simulink model "pointing_group24"  (R2023b)
settings: Solver=FixedStepAuto  StartTime=0.0  StopTime=T  RelTol=1e-3
values from neighbouring files (symbols this model uses):
  a = 6939    [Air_Drag_script.m]    (also in main.m = 6939.063; main_group24.m = 6978)
  AccMagn = 0.5    [main_group24.m]
  AccSunSens = 0.125    [main_group24.m]
  ARW = deg2rad(0.10)    [main_group24.m]
  by = 0.1    [main_group24.m]
  bz = 0.1    [main_group24.m]
  c = 2.99792*10^8    (= 299792000)    [main.m]    (also in main_group24.m = 299792458)
  Cd = 2.2    [main_group24.m]
  e = 0    [Air_Drag_script.m]    (also in main.m = 0.001304; main_group24.m)
  G = [gn, gm, gvali, gsvi]    [main.m]    (also in main_group24.m)
  GyroSampleRate = 10    [main_group24.m]
  H = [hn, hm, hvali, hsvi]    [main.m]    (also in main_group24.m)
  H_0 = ((g1_0^2)+(g1_1^2)+(h1_1^2))^0.5    (= 2.98059244128e-05)    [main_group24.m]
  i = deg2rad(97.5307)    [Air_Drag_script.m]    (also in main.m; main_group24.m = deg2rad(98))
  I_tot = [Ix 0 0; 0 Iy 0; 0 0 Iz]    [data_mass.m]    (also in main_group24.m)
  invI_tot = inv(I_tot)    [data_mass.m]    (also in main_group24.m)
  Ix = J(1,1)    [Air_Drag_script.m]    (also in data_mass.m = 0.0755003333333; main.m = 0.057749855; main_group24.m = 0.0755003333333)
  Iy = J(2,2)    [Air_Drag_script.m]    (also in data_mass.m = 0.0755003333333; main.m = 0.04143542; main_group24.m = 0.0755003333333)
  Iz = J(3,3)    [Air_Drag_script.m]    (also in data_mass.m = 0.055; main.m = 0.024624309; main_group24.m = 0.055)
  k1 = 5e-2    (= 0.05)    [main_group24.m]
  k2 = 2.5e-2    (= 0.025)    [main_group24.m]
  m = [0.1; 0.1; 0.1]    [main.m]    (also in main_group24.m)
  MB = [4; 0.1; 0.1; 0.3]    [main.m]    (also in main_group24.m)
  MMnoise = 15e-9*[1; 1; 1]    [main_group24.m]
  MMSampleRate = 1    [main_group24.m]
  mu = 3.98600433e+5    (= 398600.433)    [main.m]    (also in main_group24.m)
  n = 0.0011    [Air_Drag_script.m]    (also in main.m = sqrt(mu/a^3); main_group24.m = sqrt(mu/a^3))
  n_E = 729.2e-07    (= 7.292e-05)    [main_group24.m]
  om_E = 0.000072921    (= 7.2921e-05)    [main_group24.m]
  P = Fe/c    (= 4.52980041279e-06)    [main_group24.m]
  q0 = [ 1 1 1 1 ]'    [Air_Drag_script.m]    (also in main_group24.m = [0 0 0 1]')
  R_e = 6378    [main.m]    (also in main_group24.m)
  rho_air = 1.65e-13    [Air_Drag_script.m]    (also in main_group24.m = 6.967e-13)
  rho_d_body = 0.1*2/3    (= 0.0666666666667)    [main_group24.m]
  rho_d_sp = 0.1*2/3    (= 0.0666666666667)    [main_group24.m]
  rho_s_body = 0.5    [main_group24.m]
  rho_s_sp = 0.1    [main_group24.m]
  RRW = deg2rad(0.3)    [main_group24.m]
  SP = [1; 0.3; 0.1; 0.01]    [main.m]    (also in main_group24.m = [0.25; 0.1; 0.3; 0.01])
undefined symbols (not defined in the file or in its folder): pan, s1, s2, s3, s4, s5, s6, thrust
libraries: vrlib x25, matrix_library x17, simulink_extras x8, sharedutil x3, simulink x1
(part 5 of 5)

== system pointing_group24/Desturbances/External Torques/Solar radiation/Torque arm MB/creazione raggi vettore tra CM MB e centro facce illuminate della faccia che ha come normale l'asse i/If Action Subsystem3 ==
  Action Port : ActionPort  ActionPortLabel=else
  Constant : Constant  Value=[0;0;0]
  Out1 : Outport
  wires:
  Constant/1 -> Out1/1

== system pointing_group24/Desturbances/External Torques/Solar radiation/Torque arm MB/creazione raggi vettore tra CM MB e centro facce illuminate della faccia che ha come normale l'asse i/If Action Subsystem4 ==
  Areas_vect : Inport
  MB : Inport  Port=2
  Action Port : ActionPort  ActionPortLabel=if(u1<0 & u2>0)
  Add : Sum  Inputs=+|-
  Add1 : Sum  Inputs=+|-
  Add2 : Sum
  Demux : Demux  Outputs=3
  Demux2 : Demux
  Divide : Product  Inputs=*/
  Divide1 : Product  Inputs=*/
  Gain{,1..3} (4 alike) : Gain  Gain=1/2
  Gain4 : Gain  Gain=-1
  Ground : Ground
  Ground1 : Ground
  Mux : Mux  Inputs=3
  Mux1 : Mux  Inputs=3
  Reshape : Reshape  OutputDimensionality=Column vector (2-D)
  Reshape2 : Reshape  OutputDimensionality=Column vector (2-D)
  Reshape3 : Reshape  OutputDimensionality=Column vector (2-D)
  Terminator{1..2,8..9} (4 alike) : Terminator
  r_cface_cluce_zneg_y_pos : Outport
  wires:
  [h_MB] -> Divide1/2
  [b_MB] -> Gain2/1
  Add1/1 -> Mux1/2
  Gain4/1 -> Mux/3
  Add/1 -> Gain4/1
  [h_MB] -> Gain/1
  [b_MB] -> Divide/2
  Divide/1 -> Gain1/1
  Mux/1 -> Reshape2/1  "raggio vettore che collega il centro geom della faccia con il centro geom della faccia illuminata dal sole lungo -k"
  Gain1/1 -> Add/2
  Gain/1 -> Add/1
  Areas_vect/1 -> Reshape/1
  Ground1/1 -> Mux/1, Mux/2
  Reshape/1 -> Demux/1
  Mux1/1 -> Reshape3/1  "raggio vettore che collega il centro geom della faccia con il centro geom della faccia illuminata dal sole lungo j"
  Ground/1 -> Mux1/3, Mux1/1
  Gain3/1 -> Add1/2
  Gain2/1 -> Add1/1
  Divide1/1 -> Gain3/1
  Reshape2/1 -> Add2/1
  Reshape3/1 -> Add2/2
  Add2/1 -> r_cface_cluce_zneg_y_pos/1
  Demux/2 -> Terminator9/1
  Demux/3 -> Terminator8/1
  Demux/1 -> Divide1/1, Divide/1
  Demux2/1 -> Terminator2/1
  Demux2/2 -> Terminator1/1
  MB/1 -> Demux2/1
  Demux2/3 -> [b_MB]
  Demux2/4 -> [h_MB]

== system pointing_group24/Desturbances/External Torques/Solar radiation/Torque arm MB/creazione raggi vettore tra CM MB e centro facce illuminate della faccia che ha come normale l'asse i/If Action Subsystem5 ==
  Action Port : ActionPort  ActionPortLabel=else
  Constant : Constant  Value=[0;0;0]
  Out1 : Outport
  wires:
  Constant/1 -> Out1/1

== system pointing_group24/Desturbances/External Torques/Solar radiation/Torque arm MB/creazione raggi vettore tra CM MB e centro facce illuminate della faccia che ha come normale l'asse i/If Action Subsystem6 ==
  Action Port : ActionPort  ActionPortLabel=else
  Constant : Constant  Value=[0;0;0]
  Out1 : Outport
  wires:
  Constant/1 -> Out1/1

== system pointing_group24/Desturbances/External Torques/Solar radiation/Torque arm MB/creazione raggi vettore tra CM MB e centro facce illuminate della faccia che ha come normale l'asse i/If Action Subsystem8 ==
  Action Port : ActionPort  ActionPortLabel=else
  Constant : Constant  Value=[0;0;0]
  Out1 : Outport
  wires:
  Constant/1 -> Out1/1

== system pointing_group24/Desturbances/External Torques/Solar radiation/Torque arm MB/creazione raggi vettore tra CM MB e centro facce illuminate della faccia che ha come normale l'asse i/creating distance between cm MB and centro geom lato ==
  MB : Inport
  pointer : Inport  Port=2
  Demux : Demux
  Gain : Gain  Gain=1/2
  Ground : Ground
  Mux : Mux  Inputs=3
  Product : Product
  Reshape : Reshape  OutputDimensionality=Column vector (2-D)
  Terminator : Terminator
  Terminator1 : Terminator
  Terminator3 : Terminator
  Out1 : Outport
  wires:
  Reshape/1 -> Out1/1
  Mux/1 -> Reshape/1
  MB/1 -> Demux/1
  Demux/1 -> Terminator/1
  Demux/2 -> Terminator1/1
  Ground/1 -> Mux/3, Mux/1
  Demux/4 -> Terminator3/1
  Demux/3 -> Gain/1
  Product/1 -> Mux/2
  pointer/1 -> Product/2
  Gain/1 -> Product/1

== system pointing_group24/Desturbances/External Torques/Solar radiation/Torque arm MB/creazione raggi vettore tra CM MB e centro facce illuminate della faccia che ha come normale l'asse j/If Action Subsystem ==
  Areas_vect : Inport
  MB : Inport  Port=2
  Action Port : ActionPort  ActionPortLabel=if(u1>0 & u2>0)
  Add : Sum  Inputs=+|-
  Add1 : Sum  Inputs=+|-
  Add2 : Sum
  Demux : Demux  Outputs=3
  Demux2 : Demux
  Divide : Product  Inputs=*/
  Divide1 : Product  Inputs=*/
  Gain{,1..3} (4 alike) : Gain  Gain=1/2
  Ground : Ground
  Ground1 : Ground
  Mux : Mux  Inputs=3
  Mux1 : Mux  Inputs=3
  Reshape : Reshape  OutputDimensionality=Column vector (2-D)
  Reshape2 : Reshape  OutputDimensionality=Column vector (2-D)
  Reshape3 : Reshape  OutputDimensionality=Column vector (2-D)
  Terminator{1..2,8..9} (4 alike) : Terminator
  r_cface_cluce_xz_pos : Outport
  wires:
  Add/1 -> Mux/3
  Divide/1 -> Gain1/1
  Mux/1 -> Reshape2/1  "raggio vettore che collega il centro geom della faccia con il centro geom della faccia illuminata dal sole lungo k"
  Gain1/1 -> Add/2
  Demux/2 -> Divide1/1, Divide/1
  [h_MB] -> Gain/1
  Gain/1 -> Add/1
  [a_MB] -> Divide/2
  Areas_vect/1 -> Reshape/1
  Ground1/1 -> Mux/2, Mux/1
  Reshape/1 -> Demux/1
  Add1/1 -> Mux1/1
  [h_MB] -> Divide1/2
  Mux1/1 -> Reshape3/1  "raggio vettore che collega il centro geom della faccia con il centro geom della faccia illuminata dal sole lungo i"
  Ground/1 -> Mux1/2, Mux1/3
  Gain3/1 -> Add1/2
  Gain2/1 -> Add1/1
  Divide1/1 -> Gain3/1
  [a_MB] -> Gain2/1
  Reshape2/1 -> Add2/1
  Reshape3/1 -> Add2/2
  Add2/1 -> r_cface_cluce_xz_pos/1
  Demux/1 -> Terminator9/1
  Demux/3 -> Terminator8/1
  Demux2/1 -> Terminator2/1
  Demux2/2 -> [a_MB]
  MB/1 -> Demux2/1
  Demux2/3 -> Terminator1/1
  Demux2/4 -> [h_MB]

== system pointing_group24/Desturbances/External Torques/Solar radiation/Torque arm MB/creazione raggi vettore tra CM MB e centro facce illuminate della faccia che ha come normale l'asse j/If Action Subsystem1 ==
  Areas_vect : Inport
  MB : Inport  Port=2
  Action Port : ActionPort  ActionPortLabel=if(u1<0 & u2>0)
  Add : Sum  Inputs=+|-
  Add1 : Sum  Inputs=+|-
  Add2 : Sum
  Demux : Demux  Outputs=3
  Demux2 : Demux
  Divide : Product  Inputs=*/
  Divide1 : Product  Inputs=*/
  Gain{,1..3} (4 alike) : Gain  Gain=1/2
  Gain4 : Gain  Gain=-1
  Ground : Ground
  Ground1 : Ground
  Mux : Mux  Inputs=3
  Mux1 : Mux  Inputs=3
  Reshape : Reshape  OutputDimensionality=Column vector (2-D)
  Reshape2 : Reshape  OutputDimensionality=Column vector (2-D)
  Reshape3 : Reshape  OutputDimensionality=Column vector (2-D)
  Terminator{1..2,8..9} (4 alike) : Terminator
  r_cface_cluce_x_pos_z_neg : Outport
  wires:
  Demux/3 -> Terminator8/1
  Demux/1 -> Terminator9/1
  Add2/1 -> r_cface_cluce_x_pos_z_neg/1
  Reshape3/1 -> Add2/2
  Reshape2/1 -> Add2/1
  [a_MB] -> Gain2/1
  Divide1/1 -> Gain3/1
  Gain2/1 -> Add1/1
  Gain3/1 -> Add1/2
  Ground/1 -> Mux1/3, Mux1/2
  Mux1/1 -> Reshape3/1  "raggio vettore che collega il centro geom della faccia con il centro geom della faccia illuminata dal sole lungo i"
  [h_MB] -> Divide1/2
  Add1/1 -> Mux1/1
  Reshape/1 -> Demux/1
  Ground1/1 -> Mux/1, Mux/2
  Areas_vect/1 -> Reshape/1
  [a_MB] -> Divide/2
  Gain/1 -> Add/1
  [h_MB] -> Gain/1
  Demux/2 -> Divide/1, Divide1/1
  Gain1/1 -> Add/2
  Mux/1 -> Reshape2/1  "raggio vettore che collega il centro geom della faccia con il centro geom della faccia illuminata dal sole lungo -k"
  Divide/1 -> Gain1/1
  Add/1 -> Gain4/1
  Gain4/1 -> Mux/3
  Demux2/1 -> Terminator2/1
  Demux2/2 -> [a_MB]
  MB/1 -> Demux2/1
  Demux2/3 -> Terminator1/1
  Demux2/4 -> [h_MB]

== system pointing_group24/Desturbances/External Torques/Solar radiation/Torque arm MB/creazione raggi vettore tra CM MB e centro facce illuminate della faccia che ha come normale l'asse j/If Action Subsystem2 ==
  Areas_vect : Inport
  MB : Inport  Port=2
  Action Port : ActionPort  ActionPortLabel=if(u1>0 & u2<0)
  Add : Sum  Inputs=+|-
  Add1 : Sum  Inputs=+|-
  Add2 : Sum
  Demux : Demux  Outputs=3
  Demux2 : Demux
  Divide : Product  Inputs=*/
  Divide1 : Product  Inputs=*/
  Gain{,1..3} (4 alike) : Gain  Gain=1/2
  Gain4 : Gain  Gain=-1
  Ground : Ground
  Ground1 : Ground
  Mux : Mux  Inputs=3
  Mux1 : Mux  Inputs=3
  Reshape : Reshape  OutputDimensionality=Column vector (2-D)
  Reshape2 : Reshape  OutputDimensionality=Column vector (2-D)
  Reshape3 : Reshape  OutputDimensionality=Column vector (2-D)
  Terminator{1..2,8..9} (4 alike) : Terminator
  r_cface_cluce_x_neg_z_pos : Outport
  wires:
  Add/1 -> Mux/3
  Divide/1 -> Gain1/1
  Mux/1 -> Reshape2/1  "raggio vettore che collega il centro geom della faccia con il centro geom della faccia illuminata dal sole lungo k"
  Gain1/1 -> Add/2
  Demux/2 -> Divide1/1, Divide/1
  [h_MB] -> Gain/1
  Gain/1 -> Add/1
  [a_MB] -> Divide/2
  Areas_vect/1 -> Reshape/1
  Ground1/1 -> Mux/2, Mux/1
  Reshape/1 -> Demux/1
  [h_MB] -> Divide1/2
  Mux1/1 -> Reshape3/1  "raggio vettore che collega il centro geom della faccia con il centro geom della faccia illuminata dal sole lungo -i"
  Ground/1 -> Mux1/2, Mux1/3
  Gain3/1 -> Add1/2
  Gain2/1 -> Add1/1
  Divide1/1 -> Gain3/1
  [a_MB] -> Gain2/1
  Reshape2/1 -> Add2/1
  Reshape3/1 -> Add2/2
  Add2/1 -> r_cface_cluce_x_neg_z_pos/1
  Demux/1 -> Terminator9/1
  Demux/3 -> Terminator8/1
  Gain4/1 -> Mux1/1
  Add1/1 -> Gain4/1
  Demux2/1 -> Terminator2/1
  Demux2/2 -> [a_MB]
  MB/1 -> Demux2/1
  Demux2/3 -> Terminator1/1
  Demux2/4 -> [h_MB]

== system pointing_group24/Desturbances/External Torques/Solar radiation/Torque arm MB/creazione raggi vettore tra CM MB e centro facce illuminate della faccia che ha come normale l'asse j/If Action Subsystem3 ==
  Areas_vect : Inport
  MB : Inport  Port=2
  Action Port : ActionPort  ActionPortLabel=if(u1<0 & u2<0)
  Add : Sum  Inputs=+|-
  Add1 : Sum  Inputs=+|-
  Add2 : Sum
  Demux : Demux  Outputs=3
  Demux2 : Demux
  Divide : Product  Inputs=*/
  Divide1 : Product  Inputs=*/
  Gain{,1..3} (4 alike) : Gain  Gain=1/2
  Gain4 : Gain  Gain=-1
  Gain5 : Gain  Gain=-1
  Ground : Ground
  Ground1 : Ground
  Mux : Mux  Inputs=3
  Mux1 : Mux  Inputs=3
  Reshape : Reshape  OutputDimensionality=Column vector (2-D)
  Reshape2 : Reshape  OutputDimensionality=Column vector (2-D)
  Reshape3 : Reshape  OutputDimensionality=Column vector (2-D)
  Terminator{1..2,8..9} (4 alike) : Terminator
  r_cface_cluce_x_neg_z_neg : Outport
  wires:
  Add1/1 -> Gain4/1
  Gain4/1 -> Mux1/1
  Demux/3 -> Terminator8/1
  Demux/1 -> Terminator9/1
  Add2/1 -> r_cface_cluce_x_neg_z_neg/1
  Reshape3/1 -> Add2/2
  Reshape2/1 -> Add2/1
  [a_MB] -> Gain2/1
  Divide1/1 -> Gain3/1
  Gain2/1 -> Add1/1
  Gain3/1 -> Add1/2
  Ground/1 -> Mux1/3, Mux1/2
  Mux1/1 -> Reshape3/1  "raggio vettore che collega il centro geom della faccia con il centro geom della faccia illuminata dal sole lungo -i"
  [h_MB] -> Divide1/2
  Reshape/1 -> Demux/1
  Ground1/1 -> Mux/1, Mux/2
  Areas_vect/1 -> Reshape/1
  [a_MB] -> Divide/2
  Gain/1 -> Add/1
  [h_MB] -> Gain/1
  Demux/2 -> Divide/1, Divide1/1
  Gain1/1 -> Add/2
  Mux/1 -> Reshape2/1  "raggio vettore che collega il centro geom della faccia con il centro geom della faccia illuminata dal sole lungo -k"
  Divide/1 -> Gain1/1
  Add/1 -> Gain5/1
  Gain5/1 -> Mux/3
  Demux2/1 -> Terminator2/1
  Demux2/2 -> [a_MB]
  MB/1 -> Demux2/1
  Demux2/3 -> Terminator1/1
  Demux2/4 -> [h_MB]

== system pointing_group24/Desturbances/External Torques/Solar radiation/Torque arm MB/creazione raggi vettore tra CM MB e centro facce illuminate della faccia che ha come normale l'asse j/If Action Subsystem4 ==
  Action Port : ActionPort  ActionPortLabel=else
  Constant : Constant  Value=[0;0;0]
  Out1 : Outport
  wires:
  Constant/1 -> Out1/1

== system pointing_group24/Desturbances/External Torques/Solar radiation/Torque arm MB/creazione raggi vettore tra CM MB e centro facce illuminate della faccia che ha come normale l'asse j/If Action Subsystem5 ==
  Action Port : ActionPort  ActionPortLabel=else
  Constant : Constant  Value=[0;0;0]
  Out1 : Outport
  wires:
  Constant/1 -> Out1/1

== system pointing_group24/Desturbances/External Torques/Solar radiation/Torque arm MB/creazione raggi vettore tra CM MB e centro facce illuminate della faccia che ha come normale l'asse j/If Action Subsystem6 ==
  Action Port : ActionPort  ActionPortLabel=else
  Constant : Constant  Value=[0;0;0]
  Out1 : Outport
  wires:
  Constant/1 -> Out1/1

== system pointing_group24/Desturbances/External Torques/Solar radiation/Torque arm MB/creazione raggi vettore tra CM MB e centro facce illuminate della faccia che ha come normale l'asse j/If Action Subsystem7 ==
  Action Port : ActionPort  ActionPortLabel=else
  Constant : Constant  Value=[0;0;0]
  Out1 : Outport
  wires:
  Constant/1 -> Out1/1

== system pointing_group24/Desturbances/External Torques/Solar radiation/Torque arm MB/creazione raggi vettore tra CM MB e centro facce illuminate della faccia che ha come normale l'asse j/creating distance between cm MB and centro geom lato1 ==
  MB : Inport
  pointer : Inport  Port=2
  Demux : Demux
  Gain : Gain  Gain=1/2
  Ground : Ground
  Mux : Mux  Inputs=3
  Product : Product
  Reshape : Reshape  OutputDimensionality=Column vector (2-D)
  Terminator : Terminator
  Terminator1 : Terminator
  Terminator2 : Terminator
  Out1 : Outport
  wires:
  Reshape/1 -> Out1/1
  Mux/1 -> Reshape/1
  MB/1 -> Demux/1
  Demux/1 -> Terminator/1
  Demux/2 -> Terminator1/1
  Demux/3 -> Terminator2/1
  Ground/1 -> Mux/2, Mux/1
  Demux/4 -> Gain/1
  pointer/1 -> Product/2
  Product/1 -> Mux/3
  Gain/1 -> Product/1

== system pointing_group24/Desturbances/External Torques/Solar radiation/Torque arm MB/creazione raggi vettore tra CM MB e centro facce illuminate della faccia che ha come normale l'asse k/If Action Subsystem ==
  Areas_vect : Inport
  MB : Inport  Port=2
  Action Port : ActionPort  ActionPortLabel=if(u1>0 & u2>0)
  Add : Sum  Inputs=+|-
  Add1 : Sum  Inputs=+|-
  Add2 : Sum
  Demux : Demux  Outputs=3
  Demux1 : Demux  Outputs=3
  Demux2 : Demux
  Divide : Product  Inputs=*/
  Divide1 : Product  Inputs=*/
  Gain{,1..3} (4 alike) : Gain  Gain=1/2
  Ground : Ground
  Ground1 : Ground
  Mux : Mux  Inputs=3
  Mux1 : Mux  Inputs=3
  Reshape{,1..3} (4 alike) : Reshape  OutputDimensionality=Column vector (2-D)
  Terminator{,1..3,8..9} (6 alike) : Terminator
  r_cface_cluce_xy_pos : Outport
  wires:
  Add/1 -> Mux/2
  Divide/1 -> Gain1/1
  Mux/1 -> Reshape2/1  "raggio vettore che collega il centro geom della faccia con il centro geom della faccia illuminata dal sole lungo j"
  Gain1/1 -> Add/2
  Demux/3 -> Divide/1
  [b_MB] -> Gain/1
  Gain/1 -> Add/1
  [a_MB] -> Divide/2
  Areas_vect/1 -> Reshape/1, Reshape1/1
  Ground1/1 -> Mux/1, Mux/3
  Reshape/1 -> Demux/1
  Add1/1 -> Mux1/1
  [b_MB] -> Divide1/2
  Mux1/1 -> Reshape3/1  "raggio vettore che collega il centro geom della faccia con il centro geom della faccia illuminata dal sole lungo x"
  Ground/1 -> Mux1/2, Mux1/3
  Demux1/3 -> Divide1/1
  Gain3/1 -> Add1/2
  Gain2/1 -> Add1/1
  Reshape1/1 -> Demux1/1
  Divide1/1 -> Gain3/1
  [a_MB] -> Gain2/1
  Reshape2/1 -> Add2/1
  Reshape3/1 -> Add2/2
  Add2/1 -> r_cface_cluce_xy_pos/1
  Demux1/1 -> Terminator/1
  Demux1/2 -> Terminator1/1
  Demux/1 -> Terminator9/1
  Demux/2 -> Terminator8/1
  MB/1 -> Demux2/1
  Demux2/1 -> Terminator2/1
  Demux2/2 -> [a_MB]
  Demux2/3 -> [b_MB]
  Demux2/4 -> Terminator3/1

== system pointing_group24/Desturbances/External Torques/Solar radiation/Torque arm MB/creazione raggi vettore tra CM MB e centro facce illuminate della faccia che ha come normale l'asse k/If Action Subsystem1 ==
  Areas_vect : Inport
  MB : Inport  Port=2
  Action Port : ActionPort  ActionPortLabel=if(u1>0 & u2<0)
  Add : Sum  Inputs=+|-
  Add1 : Sum  Inputs=+|-
  Add2 : Sum
  Demux : Demux  Outputs=3
  Demux1 : Demux  Outputs=3
  Demux2 : Demux
  Divide : Product  Inputs=*/
  Divide1 : Product  Inputs=*/
  Gain{,1..3} (4 alike) : Gain  Gain=1/2
  Gain4 : Gain  Gain=-1
  Ground : Ground
  Ground1 : Ground
  Mux : Mux  Inputs=3
  Mux1 : Mux  Inputs=3
  Reshape{,1..3} (4 alike) : Reshape  OutputDimensionality=Column vector (2-D)
  Terminator{,1..3,8..9} (6 alike) : Terminator
  r_cface_cluce_xpos_y_neg : Outport
  wires:
  Add/1 -> Gain4/1
  Divide/1 -> Gain1/1
  Mux/1 -> Reshape2/1  "raggio vettore che collega il centro geom della faccia con il centro geom della faccia illuminata dal sole lungo -j"
  Gain1/1 -> Add/2
  Demux/3 -> Divide/1
  Gain/1 -> Add/1
  Areas_vect/1 -> Reshape/1, Reshape1/1
  Ground1/1 -> Mux/1, Mux/3
  Reshape/1 -> Demux/1
  Mux1/1 -> Reshape3/1  "raggio vettore che collega il centro geom della faccia con il centro geom della faccia illuminata dal sole lungo i"
  Ground/1 -> Mux1/2, Mux1/3
  Demux1/3 -> Divide1/1
  Gain3/1 -> Add1/2
  Gain2/1 -> Add1/1
  Reshape1/1 -> Demux1/1
  Divide1/1 -> Gain3/1
  Reshape2/1 -> Add2/1
  Reshape3/1 -> Add2/2
  Add2/1 -> r_cface_cluce_xpos_y_neg/1
  Demux1/1 -> Terminator/1
  Demux1/2 -> Terminator1/1
  Demux/1 -> Terminator9/1
  Demux/2 -> Terminator8/1
  Gain4/1 -> Mux/2
  [a_MB] -> Divide/2
  [b_MB] -> Gain/1
  Add1/1 -> Mux1/1
  [b_MB] -> Divide1/2
  [a_MB] -> Gain2/1
  Demux2/1 -> Terminator2/1
  Demux2/2 -> [a_MB]
  MB/1 -> Demux2/1
  Demux2/3 -> [b_MB]
  Demux2/4 -> Terminator3/1

== system pointing_group24/Desturbances/External Torques/Solar radiation/Torque arm MB/creazione raggi vettore tra CM MB e centro facce illuminate della faccia che ha come normale l'asse k/If Action Subsystem2 ==
  Areas_vect : Inport
  MB1 : Inport  Port=2
  Action Port : ActionPort  ActionPortLabel=if(u1<0 & u2<0)
  Add : Sum  Inputs=+|-
  Add1 : Sum  Inputs=+|-
  Add2 : Sum
  Demux : Demux  Outputs=3
  Demux1 : Demux  Outputs=3
  Demux2 : Demux
  Divide : Product  Inputs=*/
  Divide1 : Product  Inputs=*/
  Gain{,1..3} (4 alike) : Gain  Gain=1/2
  Gain4 : Gain  Gain=-1
  Gain5 : Gain  Gain=-1
  Ground : Ground
  Ground1 : Ground
  Mux : Mux  Inputs=3
  Mux1 : Mux  Inputs=3
  Reshape{,1..3} (4 alike) : Reshape  OutputDimensionality=Column vector (2-D)
  Terminator{,1..3,8..9} (6 alike) : Terminator
  r_cface_cluce_xneg_y_neg : Outport
  wires:
  [a_MB] -> Divide1/2
  [b_MB] -> Gain2/1
  Add1/1 -> Gain5/1
  Gain4/1 -> Mux/1
  Add/1 -> Gain4/1
  [a_MB] -> Gain/1
  [b_MB] -> Divide/2
  Divide/1 -> Gain1/1
  Mux/1 -> Reshape2/1  "raggio vettore che collega il centro geom della faccia con il centro geom della faccia illuminata dal sole lungo -i"
  Gain1/1 -> Add/2
  Demux/3 -> Divide/1
  Gain/1 -> Add/1
  Areas_vect/1 -> Reshape/1, Reshape1/1
  Ground1/1 -> Mux/3, Mux/2
  Reshape/1 -> Demux/1
  Mux1/1 -> Reshape3/1  "raggio vettore che collega il centro geom della faccia con il centro geom della faccia illuminata dal sole lungo -j"
  Ground/1 -> Mux1/3, Mux1/1
  Demux1/3 -> Divide1/1
  Gain3/1 -> Add1/2
  Gain2/1 -> Add1/1
  Reshape1/1 -> Demux1/1
  Divide1/1 -> Gain3/1
  Reshape2/1 -> Add2/1
  Reshape3/1 -> Add2/2
  Add2/1 -> r_cface_cluce_xneg_y_neg/1
  Demux1/1 -> Terminator/1
  Demux1/2 -> Terminator1/1
  Demux/1 -> Terminator9/1
  Demux/2 -> Terminator8/1
  Gain5/1 -> Mux1/2
  Demux2/1 -> Terminator2/1
  Demux2/2 -> [a_MB]
  MB1/1 -> Demux2/1
  Demux2/3 -> [b_MB]
  Demux2/4 -> Terminator3/1

== system pointing_group24/Desturbances/External Torques/Solar radiation/Torque arm MB/creazione raggi vettore tra CM MB e centro facce illuminate della faccia che ha come normale l'asse k/If Action Subsystem3 ==
  Action Port : ActionPort  ActionPortLabel=else
  Constant : Constant  Value=[0;0;0]
  Out1 : Outport
  wires:
  Constant/1 -> Out1/1

== system pointing_group24/Desturbances/External Torques/Solar radiation/Torque arm MB/creazione raggi vettore tra CM MB e centro facce illuminate della faccia che ha come normale l'asse k/If Action Subsystem4 ==
  Areas_vect : Inport
  MB1 : Inport  Port=2
  Action Port : ActionPort  ActionPortLabel=if(u1<0 & u2>0)
  Add : Sum  Inputs=+|-
  Add1 : Sum  Inputs=+|-
  Add2 : Sum
  Demux : Demux  Outputs=3
  Demux1 : Demux  Outputs=3
  Demux2 : Demux
  Divide : Product  Inputs=*/
  Divide1 : Product  Inputs=*/
  Gain{,1..3} (4 alike) : Gain  Gain=1/2
  Gain4 : Gain  Gain=-1
  Ground : Ground
  Ground1 : Ground
  Mux : Mux  Inputs=3
  Mux1 : Mux  Inputs=3
  Reshape{,1..3} (4 alike) : Reshape  OutputDimensionality=Column vector (2-D)
  Terminator{,1..3,8..9} (6 alike) : Terminator
  r_cface_cluce_xneg_y_pos : Outport
  wires:
  Demux/2 -> Terminator8/1
  Demux/1 -> Terminator9/1
  Demux1/2 -> Terminator1/1
  Demux1/1 -> Terminator/1
  Add2/1 -> r_cface_cluce_xneg_y_pos/1
  Reshape3/1 -> Add2/2
  Reshape2/1 -> Add2/1
  Divide1/1 -> Gain3/1
  Reshape1/1 -> Demux1/1
  Gain2/1 -> Add1/1
  Gain3/1 -> Add1/2
  Demux1/3 -> Divide1/1
  Ground/1 -> Mux1/1, Mux1/3
  Mux1/1 -> Reshape3/1  "raggio vettore che collega il centro geom della faccia con il centro geom della faccia illuminata dal sole lungo j"
  Reshape/1 -> Demux/1
  Ground1/1 -> Mux/2, Mux/3
  Areas_vect/1 -> Reshape1/1, Reshape/1
  Gain/1 -> Add/1
  Demux/3 -> Divide/1
  Gain1/1 -> Add/2
  Mux/1 -> Reshape2/1  "raggio vettore che collega il centro geom della faccia con il centro geom della faccia illuminata dal sole lungo -i"
  Divide/1 -> Gain1/1
  [b_MB] -> Divide/2
  [a_MB] -> Gain/1
  Add/1 -> Gain4/1
  Gain4/1 -> Mux/1
  Add1/1 -> Mux1/2
  [b_MB] -> Gain2/1
  [a_MB] -> Divide1/2
  Demux2/1 -> Terminator2/1
  Demux2/2 -> [a_MB]
  MB1/1 -> Demux2/1
  Demux2/3 -> [b_MB]
  Demux2/4 -> Terminator3/1

== system pointing_group24/Desturbances/External Torques/Solar radiation/Torque arm MB/creazione raggi vettore tra CM MB e centro facce illuminate della faccia che ha come normale l'asse k/If Action Subsystem5 ==
  Action Port : ActionPort  ActionPortLabel=else
  Constant : Constant  Value=[0;0;0]
  Out1 : Outport
  wires:
  Constant/1 -> Out1/1

== system pointing_group24/Desturbances/External Torques/Solar radiation/Torque arm MB/creazione raggi vettore tra CM MB e centro facce illuminate della faccia che ha come normale l'asse k/If Action Subsystem6 ==
  Action Port : ActionPort  ActionPortLabel=else
  Constant : Constant  Value=[0;0;0]
  Out1 : Outport
  wires:
  Constant/1 -> Out1/1

== system pointing_group24/Desturbances/External Torques/Solar radiation/Torque arm MB/creazione raggi vettore tra CM MB e centro facce illuminate della faccia che ha come normale l'asse k/If Action Subsystem7 ==
  Action Port : ActionPort  ActionPortLabel=else
  Constant : Constant  Value=[0;0;0]
  Out1 : Outport
  wires:
  Constant/1 -> Out1/1

== system pointing_group24/Desturbances/External Torques/Solar radiation/Torque arm MB/creazione raggi vettore tra CM MB e centro facce illuminate della faccia che ha come normale l'asse k/creating distance between cm MB and centro geom lato1 ==
  MB : Inport
  pointer : Inport  Port=2
  Demux : Demux
  Gain : Gain  Gain=1/2
  Ground : Ground
  Mux : Mux  Inputs=3
  Product : Product
  Reshape : Reshape  OutputDimensionality=Column vector (2-D)
  Terminator : Terminator
  Terminator2 : Terminator
  Terminator3 : Terminator
  Out1 : Outport
  wires:
  Reshape/1 -> Out1/1
  Mux/1 -> Reshape/1
  MB/1 -> Demux/1
  Demux/1 -> Terminator/1
  Demux/3 -> Terminator2/1
  Ground/1 -> Mux/3, Mux/2
  Demux/4 -> Terminator3/1
  Product/1 -> Mux/1
  pointer/1 -> Product/2
  Demux/2 -> Gain/1
  Gain/1 -> Product/1

== system pointing_group24/Desturbances/External Torques/Solar radiation/Torque arm SP/creazione raggi vettore tra CM SP e centro di pressione della faccia illuminata/If Action Subsystem ==
  Areas_vect : Inport
  SP : Inport  Port=2
  Action Port : ActionPort  ActionPortLabel=if(u1>0 & u2>0)
  Add : Sum  Inputs=+|-
  Add1 : Sum  Inputs=+|-
  Add2 : Sum
  Demux2 : Demux
  Divide : Product  Inputs=*/
  Divide1 : Product  Inputs=*/
  Gain{,1..3} (4 alike) : Gain  Gain=1/2
  Ground : Ground
  Ground1 : Ground
  Mux : Mux  Inputs=3
  Mux1 : Mux  Inputs=3
  Reshape2 : Reshape  OutputDimensionality=Column vector (2-D)
  Reshape3 : Reshape  OutputDimensionality=Column vector (2-D)
  Terminator1 : Terminator
  Terminator2 : Terminator
  r_cface_cluce_xz_pos : Outport
  wires:
  Add/1 -> Mux/1
  Divide/1 -> Gain1/1
  Mux/1 -> Reshape2/1  "raggio vettore che collega il centro geom della faccia con il centro geom della faccia illuminata dal sole lungo i"
  Gain1/1 -> Add/2
  Areas_vect/1 -> Divide1/1, Divide/1
  [b_SP] -> Gain/1
  Gain/1 -> Add/1
  [b_SP] -> Divide/2
  Ground1/1 -> Mux/3, Mux/2
  Add1/1 -> Mux1/2
  [a_SP] -> Divide1/2
  Mux1/1 -> Reshape3/1  "raggio vettore che collega il centro geom della faccia con il centro geom della faccia illuminata dal sole lungo k"
  Ground/1 -> Mux1/1, Mux1/3
  Gain3/1 -> Add1/2
  Gain2/1 -> Add1/1
  Divide1/1 -> Gain3/1
  [a_SP] -> Gain2/1
  Reshape2/1 -> Add2/1
  Reshape3/1 -> Add2/2
  Add2/1 -> r_cface_cluce_xz_pos/1
  Demux2/1 -> Terminator2/1
  Demux2/2 -> [a_SP]
  SP/1 -> Demux2/1
  Demux2/3 -> [b_SP]
  Demux2/4 -> Terminator1/1

== system pointing_group24/Desturbances/External Torques/Solar radiation/Torque arm SP/creazione raggi vettore tra CM SP e centro di pressione della faccia illuminata/If Action Subsystem1 ==
  Areas_vect : Inport
  MB : Inport  Port=2
  Action Port : ActionPort  ActionPortLabel=if(u1<0 & u2>0)
  Add : Sum  Inputs=+|-
  Add1 : Sum  Inputs=+|-
  Add2 : Sum
  Demux2 : Demux
  Divide : Product  Inputs=*/
  Divide1 : Product  Inputs=*/
  Gain{,1..3} (4 alike) : Gain  Gain=1/2
  Ground : Ground
  Ground1 : Ground
  Mux : Mux  Inputs=3
  Mux1 : Mux  Inputs=3
  Reshape2 : Reshape  OutputDimensionality=Column vector (2-D)
  Reshape3 : Reshape  OutputDimensionality=Column vector (2-D)
  Terminator1 : Terminator
  Terminator2 : Terminator
  r_cface_cluce_x_pos_z_neg : Outport
  wires:
  Add2/1 -> r_cface_cluce_x_pos_z_neg/1
  Reshape3/1 -> Add2/2
  Reshape2/1 -> Add2/1
  [b_MB] -> Gain2/1
  Divide1/1 -> Gain3/1
  Gain2/1 -> Add1/1
  Gain3/1 -> Add1/2
  Ground/1 -> Mux1/3, Mux1/2
  Mux1/1 -> Reshape3/1  "raggio vettore che collega il centro geom della faccia con il centro geom della faccia illuminata dal sole lungo i"
  [a_MB] -> Divide1/2
  Add1/1 -> Mux1/1
  [b_MB] -> Divide/2
  Gain/1 -> Add/1
  [a_MB] -> Gain/1
  Areas_vect/1 -> Divide/1, Divide1/1
  Gain1/1 -> Add/2
  Mux/1 -> Reshape2/1  "raggio vettore che collega il centro geom della faccia con il centro geom della faccia illuminata dal sole lungo -k"
  Divide/1 -> Gain1/1
  Demux2/1 -> Terminator2/1
  Demux2/2 -> [a_MB]
  MB/1 -> Demux2/1
  Demux2/3 -> [b_MB]
  Demux2/4 -> Terminator1/1
  Add/1 -> Mux/2
  Ground1/1 -> Mux/3, Mux/1

== system pointing_group24/Desturbances/External Torques/Solar radiation/Torque arm SP/creazione raggi vettore tra CM SP e centro di pressione della faccia illuminata/If Action Subsystem2 ==
  Areas_vect : Inport
  MB : Inport  Port=2
  Action Port : ActionPort  ActionPortLabel=if(u1>0 & u2<0)
  Add : Sum  Inputs=+|-
  Add1 : Sum  Inputs=+|-
  Add2 : Sum
  Demux2 : Demux
  Divide : Product  Inputs=*/
  Divide1 : Product  Inputs=*/
  Gain{,1..3} (4 alike) : Gain  Gain=1/2
  Gain5 : Gain  Gain=-1
  Ground : Ground
  Ground1 : Ground
  Mux : Mux  Inputs=3
  Mux1 : Mux  Inputs=3
  Reshape : Reshape  OutputDimensionality=Column vector (2-D)
  Reshape2 : Reshape  OutputDimensionality=Column vector (2-D)
  Reshape3 : Reshape  OutputDimensionality=Column vector (2-D)
  Terminator1 : Terminator
  Terminator2 : Terminator
  r_cface_cluce_x_neg_z_pos : Outport
  wires:
  Add/1 -> Gain5/1
  Divide/1 -> Gain1/1
  Mux/1 -> Reshape2/1  "raggio vettore che collega il centro geom della faccia con il centro geom della faccia illuminata dal sole lungo k"
  Gain1/1 -> Add/2
  Reshape/1 -> Divide1/1, Divide/1
  [a_MB] -> Gain/1
  Gain/1 -> Add/1
  [b_MB] -> Divide/2
  Areas_vect/1 -> Reshape/1
  [a_MB] -> Divide1/2
  Mux1/1 -> Reshape3/1  "raggio vettore che collega il centro geom della faccia con il centro geom della faccia illuminata dal sole lungo -i"
  Gain3/1 -> Add1/2
  Gain2/1 -> Add1/1
  Divide1/1 -> Gain3/1
  [b_MB] -> Gain2/1
  Reshape2/1 -> Add2/1
  Reshape3/1 -> Add2/2
  Add2/1 -> r_cface_cluce_x_neg_z_pos/1
  Ground/1 -> Mux1/2, Mux1/3
  Add1/1 -> Mux1/1
  Demux2/1 -> Terminator2/1
  Demux2/2 -> [a_MB]
  MB/1 -> Demux2/1
  Demux2/3 -> [b_MB]
  Demux2/4 -> Terminator1/1
  Ground1/1 -> Mux/1, Mux/3
  Gain5/1 -> Mux/2

== system pointing_group24/Desturbances/External Torques/Solar radiation/Torque arm SP/creazione raggi vettore tra CM SP e centro di pressione della faccia illuminata/If Action Subsystem3 ==
  Areas_vect : Inport
  MB : Inport  Port=2
  Action Port : ActionPort  ActionPortLabel=if(u1<0 & u2<0)
  Add : Sum  Inputs=+|-
  Add1 : Sum  Inputs=+|-
  Add2 : Sum
  Demux2 : Demux
  Divide : Product  Inputs=*/
  Divide1 : Product  Inputs=*/
  Gain{,1..3} (4 alike) : Gain  Gain=1/2
  Gain4 : Gain  Gain=-1
  Gain5 : Gain  Gain=-1
  Ground : Ground
  Ground1 : Ground
  Mux : Mux  Inputs=3
  Mux1 : Mux  Inputs=3
  Reshape2 : Reshape  OutputDimensionality=Column vector (2-D)
  Reshape3 : Reshape  OutputDimensionality=Column vector (2-D)
  Terminator1 : Terminator
  Terminator2 : Terminator
  r_cface_cluce_x_neg_z_neg : Outport
  wires:
  Add1/1 -> Gain4/1
  Gain4/1 -> Mux1/1
  Add2/1 -> r_cface_cluce_x_neg_z_neg/1
  Reshape3/1 -> Add2/2
  Reshape2/1 -> Add2/1
  [b_MB] -> Gain2/1
  Divide1/1 -> Gain3/1
  Gain2/1 -> Add1/1
  Gain3/1 -> Add1/2
  Ground/1 -> Mux1/3, Mux1/2
  Mux1/1 -> Reshape3/1  "raggio vettore che collega il centro geom della faccia con il centro geom della faccia illuminata dal sole lungo -i"
  [a_MB] -> Divide1/2
  Ground1/1 -> Mux/3, Mux/1
  [b_MB] -> Divide/2
  Gain/1 -> Add/1
  [a_MB] -> Gain/1
  Areas_vect/1 -> Divide/1, Divide1/1
  Gain1/1 -> Add/2
  Mux/1 -> Reshape2/1  "raggio vettore che collega il centro geom della faccia con il centro geom della faccia illuminata dal sole lungo -k"
  Divide/1 -> Gain1/1
  Add/1 -> Gain5/1
  Gain5/1 -> Mux/2
  Demux2/1 -> Terminator2/1
  Demux2/2 -> [a_MB]
  MB/1 -> Demux2/1
  Demux2/3 -> [b_MB]
  Demux2/4 -> Terminator1/1

== system pointing_group24/Desturbances/External Torques/Solar radiation/Torque arm SP/creazione raggi vettore tra CM SP e centro di pressione della faccia illuminata/If Action Subsystem4 ==
  Action Port : ActionPort  ActionPortLabel=else
  Constant : Constant  Value=[0;0;0]
  Out1 : Outport
  wires:
  Constant/1 -> Out1/1

== system pointing_group24/Desturbances/External Torques/Solar radiation/Torque arm SP/creazione raggi vettore tra CM SP e centro di pressione della faccia illuminata/If Action Subsystem5 ==
  Action Port : ActionPort  ActionPortLabel=else
  Constant : Constant  Value=[0;0;0]
  Out1 : Outport
  wires:
  Constant/1 -> Out1/1

== system pointing_group24/Desturbances/External Torques/Solar radiation/Torque arm SP/creazione raggi vettore tra CM SP e centro di pressione della faccia illuminata/If Action Subsystem6 ==
  Action Port : ActionPort  ActionPortLabel=else
  Constant : Constant  Value=[0;0;0]
  Out1 : Outport
  wires:
  Constant/1 -> Out1/1

== system pointing_group24/Desturbances/External Torques/Solar radiation/Torque arm SP/creazione raggi vettore tra CM SP e centro di pressione della faccia illuminata/If Action Subsystem7 ==
  Action Port : ActionPort  ActionPortLabel=else
  Constant : Constant  Value=[0;0;0]
  Out1 : Outport
  wires:
  Constant/1 -> Out1/1

== system pointing_group24/Desturbances/External Torques/Solar radiation/Torque arm SP/creazione raggi vettore tra CM SP e centro di pressione della faccia illuminata/creating distance between cm MB and centro geom lato1 ==
  MB : Inport
  pointer : Inport  Port=2
  Demux : Demux
  Gain : Gain  Gain=1/2
  Ground : Ground
  Mux : Mux  Inputs=3
  Product : Product
  Reshape : Reshape  OutputDimensionality=Column vector (2-D)
  Terminator : Terminator
  Terminator1 : Terminator
  Terminator2 : Terminator
  Out1 : Outport
  wires:
  Reshape/1 -> Out1/1
  Mux/1 -> Reshape/1
  MB/1 -> Demux/1
  Demux/1 -> Terminator/1
  Demux/2 -> Terminator1/1
  Demux/3 -> Terminator2/1
  Ground/1 -> Mux/2, Mux/1
  Demux/4 -> Gain/1
  pointer/1 -> Product/2
  Product/1 -> Mux/3
  Gain/1 -> Product/1

== matlab function pointing_group24/Attitude Determination/Attitude Determination ==
  data: A_BN input; b_B input; q_est output; accuracy1 input; S_meas_B input; accuracy2 input
function q_est = q_method(A_BN, b_B, accuracy1, S_meas_B, accuracy2)

% Wahba's Problem: to solve the problem using a statistical method, at least 2 vector measurements 
% and the knowledge of relative precision of the sensors is needed to minimize
% the weighted error function.
% 
% INPUTS:
% A_BN [3x3] : DCM
% b_B [3x1] : vector measurement of first sensor [T]
% accuracy1 [1] : accuracy of the first sensor [deg]
% S_meas_B [3x1] : vector measurement of second sensor [km]
% accuracy2 [1] : accuracy of the second sensor [deg]

s_B1 = b_B;
s_B2 = S_meas_B;

v_N1 = A_BN' * b_B;
v_N2 = A_BN' * s_B2;

precision1 = 1/norm(accuracy1);
precision2 = 1/norm(accuracy2);

% Weights normalization
alpha1 = precision1/(precision1+precision2);
alpha2 = precision2/(precision1+precision2);

% Solve for B
B = alpha1 * s_B1 * v_N1' + alpha2 * s_B2 * v_N2';

% % Singular value decomposition
% [U,~,V] = svd(B);
% M = diag([1, 1, det(U)*det(V)]);
% A_BN_est = U*M*V';

S = B + B';
Z = [B(2,3) - B(3,2); B(3,1) - B(1,3); B(1,2) - B(2,1)];
sigma = trace(B);

K =  [ S-sigma*eye(3) Z ; Z' sigma];

[q, lambda] = eig(K);
lambda_est = [lambda(1,1) lambda(2,2) lambda(3,3) lambda(4,4)];
[m, i] = max(real(lambda_est));
q_est = real(q(:, i));

end

== matlab function pointing_group24/Attitude Determination/Attitude Determination1 ==
  data: A_BN input; b_B input; A_BN_est output; accuracy1 input; S_meas_B input; accuracy2 input
function A_BN_est = statistical_method(A_BN, b_B, accuracy1, S_meas_B, accuracy2)

% Wahba's Problem: to solve the problem using a statistical method, at least 2 vector measurements 
% and the knowledge of relative precision of the sensors is needed to minimize
% the weighted error function.
% 
% INPUTS:
% A_BN [3x3] : DCM
% b_N_m [3x1] : vector measurement of first sensor [T]
% accuracy1 [1] : accuracy of the first sensor [deg]
% r_N_m [3x1] : vector measurement of second sensor [km]
% accuracy2 [1] : accuracy of the second sensor [deg]

s_B1 = b_B;
s_B2 = S_meas_B;

v_N1 = A_BN' * b_B;
v_N2 = A_BN' * s_B2;

precision1 = 1/norm(accuracy1);
precision2 = 1/norm(accuracy2);

% Weights normalization
alpha1 = precision1/(precision1+precision2);
alpha2 = precision2/(precision1+precision2);

% Solve for B
B = alpha1 * s_B1 * v_N1' + alpha2 * s_B2 * v_N2';

% Singular value decomposition
[U,~,V] = svd(B);
M = diag([1, 1, det(U)*det(V)]);
A_BN_est = U*M*V';


end

== matlab function pointing_group24/Attitude Control/Thrusters/Ideal Control Torque/MATLAB Function2 ==
  data: S input; T output; T_min input; T_max input
function T = variableT2(S, T_min, T_max)
S = abs(S);
S_min = 3*1e-6;
S_max = 1e-3;

t = [0 0 0];

for i=1:3
    if S(i) > S_min && S(i) <= S_max
       t(i) = interp1([S_min S_max],[T_min T_max],S(i));
    elseif S(i) > S_max
        t(i) = T_max;
    elseif S(i) < S_min
        t(i) = 0;
    end
end

T = [t(1);t(2);t(3)];

== matlab function pointing_group24/Desturbances/External Torques/Magnetic field/MATLAB Function ==
  data: r_LVLH input; r input; b_N output; t input; G input; H input
function b_N  = magnet(r_LVLH, r, t, G, H)
% Inputs
% r Geocentric radius
% theta Latitude measured in degrees positive from equator
% phi Longitude measured in degrees positive east from Greenwich
%
% Outputs - magnetic field strength in local tangential coordinates
% Br B in radial direction
% Bt B in theta direction
% Bp B in phi direction

% Computing the right ascension alpha, the declination delta, the longitude lon and the co-latitude phi
r_norm = norm(r_LVLH);
delta = asin(r_LVLH(3)/r_norm);
if(r_LVLH(2)/r_norm > 0)
    alpha = acos((r_LVLH(1)/r_norm)/cos(delta));
else 
    alpha = 2*pi -  acos((r_LVLH(1)/r_norm)/cos(delta));
end
theta = -delta;
om_E = deg2rad(15.04)/3600;
Gren_lon = om_E*t;
phi = (alpha - Gren_lon);

% Checks to see if located at either pole to avoid singularities
if (theta>-0.00000001 && theta<0.00000001)
theta=0.00000001;
elseif(theta<180.00000001 && theta>179.99999999)
theta=179.99999999;
end
% The angles must be converted from degrees into radians
theta=(90-theta)*pi/180;
phi = phi*pi/180;
a=6371.2; % Reference radius used in IGRF
% This section of the code simply reads in the g and h Schmidt
% quasi-normalized coefficients
gn = G(:,1);
gm = G(:,2);
gvali = G(:,3);
hn = H(:,1);
hm = H(:,2);
hvali = H(:,3);
%[gn, gm, gvali, ~] = textread('igrfSg.txt','%f %f %f %f');
%[hn, hm, hvali, ~]= textread('igrfSh.txt','%f %f %f %f');
N=max(gn);
g=zeros(N,N+1);
h=zeros(N,N+1);
for x=1:length(gn)
g(gn(x),gm(x)+1) = gvali(x);
h(hn(x),hm(x)+1) = hvali(x);
end
% Initialize each of the variables
% Br B in the radial driection
% Bt B in the theta direction
% Bp B in the phi direction
% P The associated Legendre polynomial evaluated at cos(theta)
% The nomenclature for the recursive values generally follows
% the form P10 = P(n-1,m-0)
% dP The partial derivative of P with respect to theta
Br=0; Bt=0; Bp=0;
P11=1; P10=P11;
dP11=0; dP10=dP11;
for m=0:N
for n=1:N
if m<=n
% Calculate Legendre polynomials and derivatives recursively
if n==m
P2 = sin(theta)*P11;
dP2 = sin(theta)*dP11 + cos(theta)*P11;
P11=P2; P10=P11; P20=0;
dP11=dP2; dP10=dP11; dP20=0;
elseif n==1
P2 = cos(theta)*P10;
dP2 = cos(theta)*dP10 - sin(theta)*P10;
P20=P10; P10=P2;
dP20=dP10; dP10=dP2;
else
P20=P10;
dP20=dP10;
K = ((n-1)^2-m^2)/((2*n-1)*(2*n-3));
P2 = cos(theta)*P10 - K*P20;
dP2 = cos(theta)*dP10 - sin(theta)*P10 - K*dP20;
P10=P2;
dP10=dP2;
end
% Calculate Br, Bt, and Bp
Br = Br + (a/r)^(n+2)*(n+1)*...
((g(n,m+1)*cos(m*phi) + h(n,m+1)*sin(m*phi))*P2);
Bt = Bt + (a/r)^(n+2)*...
((g(n,m+1)*cos(m*phi) + h(n,m+1)*sin(m*phi))*dP2);
Bp = Bp + (a/r)^(n+2)*...
(m*(-g(n,m+1)*sin(m*phi) + h(n,m+1)*cos(m*phi))* P2);
end
end
end
% Spherical coordinates
Br = Br;
Bt = -Bt;
Bp = -Bp / sin(theta);

% Inertial cartesian coordinates
LST = Gren_lon + phi;
lat = theta;
Bx = (Br*cos(lat)+Bt*sin(lat))*cos(LST) - Bp*sin(LST);
By = (Br*cos(lat)+Bt*sin(lat))*sin(LST) + Bp*cos(LST);
Bz = (Br*sin(lat)+Bt*cos(lat));

b_N = [Bx; By; Bz];

end

== matlab function pointing_group24/Attitude Control/Ideal controller/MATLAB Function ==
  data: A input; Av output
function Av = inv_hat(A)

B = A' - A;
Av = [-B(2,3) B(1,3) -B(1,2)]';

== matlab function pointing_group24/Attitude Control/Thrusters/MATLAB Function2 ==
  data: u_c input; u_c_real output; th_level output; T_min input; T_max input
function [u_c_real,th_level] = thrust_level(u_c, T_min, T_max)
u_c_real = zeros(size(u_c));
th_level = zeros(size(u_c));
% T_min = 10*1e-6;
% T_max = 500*1e-6;

for i=1:length(u_c)
   if u_c(i) < T_min
       u_c_real(i) = 0;
   elseif u_c(i) >= T_max
       u_c_real(i) = T_max;
   else
       u_c_real(i) = u_c(i);
   end
   th_level(i) = u_c_real(i)*100/T_max;
end

== matlab function pointing_group24/Attitude Control/Thrusters/MATLAB Function1 ==
  data: u input; y output
function y = pseudoinverse(u)

y = pinv(u);
